simulink model "MS_AEB_201223"  (R2019b)
settings: Solver=ode1  StartTime=0.0  StopTime=inf  FixedStep=0.001  RelTol=1e-3
PreLoadFcn:
  | vehicle = 'Car'; if ~length(which('cmself')), cmenv; end
  | MS_AEB_201223_bus
InitFcn:
  | vehicle = 'Car'; if ~length(which('cmself')), cmenv; end
  | MS_AEB_201223_bus
libraries: CarMaker4SL x4
Description:
  | CarMaker Plug-in Model Target
settings Model: Creator=ambl  LastModifiedBy=ambl
settings RTWCC: Description=CarMaker Plug-in Model Target  SystemTargetFile=CarMaker.tlc  TemplateMakefile=CarMaker_unix-linux64.tmf
settings CodeAppCC: MaxIdLength=127
settings STFCustomTargetCC: TargetLangStandard=C99 (ISO)  CombineOutputUpdateFcns=on  MultiInstanceERTCode=on  CodeInterfacePackaging=Reusable function  GenerateAllocFcn=on  SystemTargetFile=CarMaker.tlc
settings GRTTargetCC: ParMdlRefBuildCompliant=off  CompOptLevelCompliant=off  ConcurrentExecutionCompliant=off  MatFileLogging=off  MultiInstanceERTCode=on  CodeInterfacePackaging=Reusable function  CPPClassGenCompliant=off  GenerateAllocFcn=on  UseToolchainInfoCompliant=off

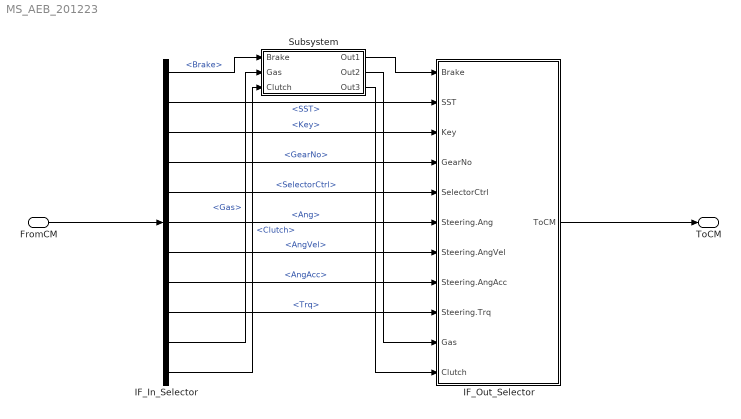
== system MS_AEB_201223 ==
  FromCM : Inport  OutDataTypeStr=Bus: cmVehicleControlIn
  IF_In_Selector : BusSelector  OutputSignals=Brake,SST,Key,GearNo,SelectorCtrl,Steering.Ang,Steering.AngVel,Steering.AngAcc,Steering.Trq,Gas,Clutch
  IF_Out_Selector : Subsystem  mask(Signal Selection){}
      mask help: Signal Selection Block
      settings: OpenFcn=cmSignalSelect('SignalSelection_CB',gcb)
  Subsystem : Subsystem
  ToCM : Outport  OutDataTypeStr=Bus: cmVehicleControlOut
  wires:
  IF_Out_Selector/1(ToCM) -> ToCM/1
  IF_In_Selector/8 -> IF_Out_Selector/8(Steering.AngAcc)  "<AngAcc>"
  FromCM/1 -> IF_In_Selector/1
  IF_In_Selector/10 -> Subsystem/2("Gas ")  "<Gas>"
  Subsystem/2(Out2) -> IF_Out_Selector/10(Gas)
  IF_In_Selector/7 -> IF_Out_Selector/7(Steering.AngVel)  "<AngVel>"
  IF_In_Selector/9 -> IF_Out_Selector/9(Steering.Trq)  "<Trq>"
  IF_In_Selector/4 -> IF_Out_Selector/4(GearNo)  "<GearNo>"
  IF_In_Selector/11 -> Subsystem/3("Clutch ")  "<Clutch>"
  Subsystem/3(Out3) -> IF_Out_Selector/11(Clutch)
  Subsystem/1(Out1) -> IF_Out_Selector/1(Brake)
  IF_In_Selector/5 -> IF_Out_Selector/5(SelectorCtrl)  "<SelectorCtrl>"
  IF_In_Selector/3 -> IF_Out_Selector/3(Key)  "<Key>"
  IF_In_Selector/1 -> Subsystem/1(Brake)  "<Brake>"
  IF_In_Selector/2 -> IF_Out_Selector/2(SST)  "<SST>"
  IF_In_Selector/6 -> IF_Out_Selector/6(Steering.Ang)  "<Ang>"

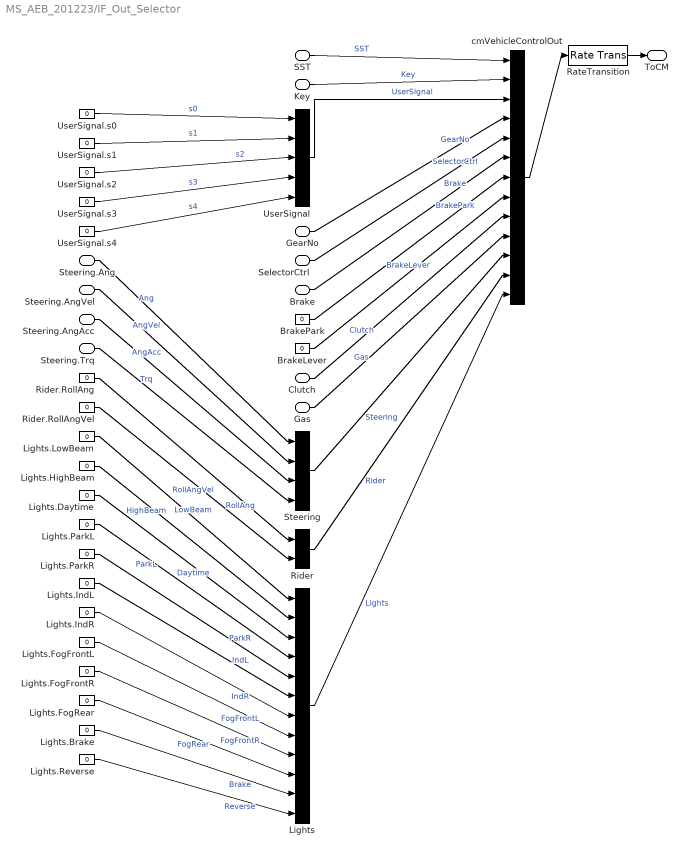
== system MS_AEB_201223/IF_Out_Selector ==
  Brake : Inport
  SST : Inport  Port=2
  Key : Inport  Port=3
  GearNo : Inport  Port=4
  SelectorCtrl : Inport  Port=5
  Steering.Ang : Inport  Port=6
  Steering.AngVel : Inport  Port=7
  Steering.AngAcc : Inport  Port=8
  Steering.Trq : Inport  Port=9
  Gas : Inport  Port=10
  Clutch : Inport  Port=11
  BrakeLever : Constant  Value=0
  BrakePark : Constant  Value=0
  Lights : BusCreator  Inputs=12
  Lights.Brake : Constant  Value=0
  Lights.Daytime : Constant  Value=0
  Lights.FogFrontL : Constant  Value=0
  Lights.FogFrontR : Constant  Value=0
  Lights.FogRear : Constant  Value=0
  Lights.HighBeam : Constant  Value=0
  Lights.IndL : Constant  Value=0
  Lights.IndR : Constant  Value=0
  Lights.LowBeam : Constant  Value=0
  Lights.ParkL : Constant  Value=0
  Lights.ParkR : Constant  Value=0
  Lights.Reverse : Constant  Value=0
  RateTransition : RateTransition  OutPortSampleTime=str2num(get_param(bdroot,'FixedStep'))
  Rider : BusCreator  Inputs=2
  Rider.RollAng : Constant  Value=0
  Rider.RollAngVel : Constant  Value=0
  Steering : BusCreator  Inputs=4
  UserSignal : BusCreator  Inputs=5
  UserSignal.s{0..4} (5 alike) : Constant  Value=0
  cmVehicleControlOut : BusCreator  Inputs=13
  ToCM : Outport
  wires:
  RateTransition/1 -> ToCM/1
  cmVehicleControlOut/1 -> RateTransition/1
  UserSignal/1 -> cmVehicleControlOut/3  "UserSignal"
  UserSignal.s0/1 -> UserSignal/1  "s0"
  UserSignal.s1/1 -> UserSignal/2  "s1"
  UserSignal.s2/1 -> UserSignal/3  "s2"
  UserSignal.s3/1 -> UserSignal/4  "s3"
  UserSignal.s4/1 -> UserSignal/5  "s4"
  BrakePark/1 -> cmVehicleControlOut/7  "BrakePark"
  BrakeLever/1 -> cmVehicleControlOut/8  "BrakeLever"
  Steering/1 -> cmVehicleControlOut/11  "Steering"
  Rider/1 -> cmVehicleControlOut/12  "Rider"
  Rider.RollAng/1 -> Rider/1  "RollAng"
  Rider.RollAngVel/1 -> Rider/2  "RollAngVel"
  Lights/1 -> cmVehicleControlOut/13  "Lights"
  Lights.LowBeam/1 -> Lights/1  "LowBeam"
  Lights.HighBeam/1 -> Lights/2  "HighBeam"
  Lights.Daytime/1 -> Lights/3  "Daytime"
  Lights.ParkL/1 -> Lights/4  "ParkL"
  Lights.ParkR/1 -> Lights/5  "ParkR"
  Lights.IndL/1 -> Lights/6  "IndL"
  Lights.IndR/1 -> Lights/7  "IndR"
  Lights.FogFrontL/1 -> Lights/8  "FogFrontL"
  Lights.FogFrontR/1 -> Lights/9  "FogFrontR"
  Lights.FogRear/1 -> Lights/10  "FogRear"
  Lights.Brake/1 -> Lights/11  "Brake"
  Lights.Reverse/1 -> Lights/12  "Reverse"
  Brake/1 -> cmVehicleControlOut/6  "Brake"
  SST/1 -> cmVehicleControlOut/1  "SST"
  Key/1 -> cmVehicleControlOut/2  "Key"
  GearNo/1 -> cmVehicleControlOut/4  "GearNo"
  SelectorCtrl/1 -> cmVehicleControlOut/5  "SelectorCtrl"
  Steering.Ang/1 -> Steering/1  "Ang"
  Steering.AngVel/1 -> Steering/2  "AngVel"
  Steering.AngAcc/1 -> Steering/3  "AngAcc"
  Steering.Trq/1 -> Steering/4  "Trq"
  Clutch/1 -> cmVehicleControlOut/9  "Clutch"
  Gas/1 -> cmVehicleControlOut/10  "Gas"

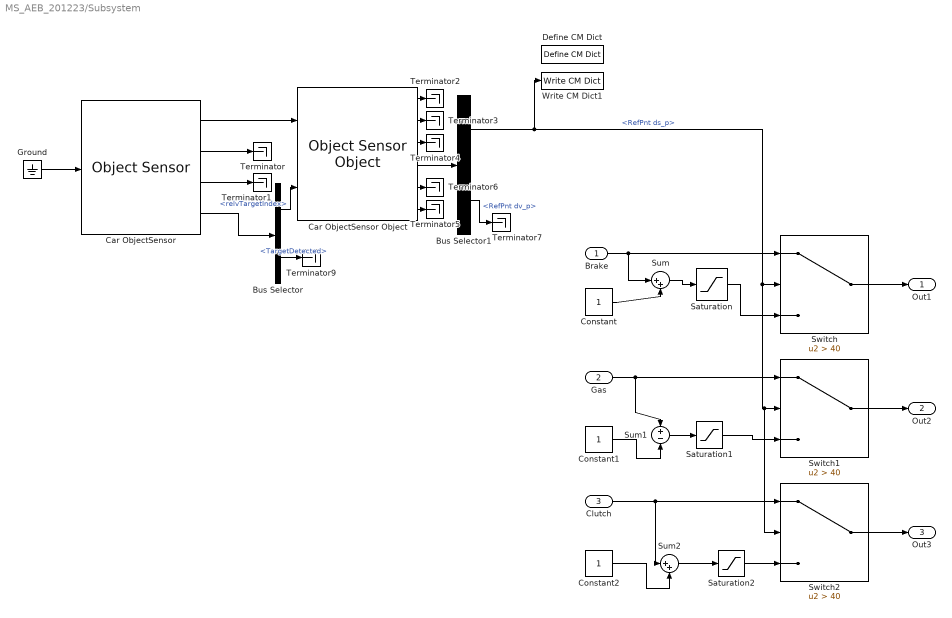
== system MS_AEB_201223/Subsystem ==
  Brake : Inport
  "Gas " : Inport  Port=2
  "Clutch " : Inport  Port=3
  Bus Selector : BusSelector  OutputSignals=relvTargetIndex,TargetDetected
  Bus Selector1 : BusSelector  OutputSignals=RefPnt ds_p,RefPnt dv_p
  Car ObjectSensor : CarMaker4SL/Sensors/Object Sensor  xname=OB00  xstime=Continuous
      settings: SourceProductName=CarMaker4SL
  Car ObjectSensor Object : CarMaker4SL/Sensors/Object Sensor Object  xname=INPORT  ximode=World Objects  xstime=Continuous
      settings: SourceProductName=CarMaker4SL
  Constant : Constant
  Constant1 : Constant
  Constant2 : Constant
  Define CM Dict : CarMaker4SL/Define CM Dict  xname=MS_Quant  xmono=off  xtype=Double4  xdvaplace=None  xnstates=0  xfirststate=0  xinitial=0
  Ground : Ground
  Saturation : Saturate  UpperLimit=1  LowerLimit=0
  Saturation1 : Saturate  UpperLimit=1  LowerLimit=0
  Saturation2 : Saturate  UpperLimit=1  LowerLimit=0
  Sum : Sum  Inputs=|++
  Sum1 : Sum  Inputs=+-
  Sum2 : Sum  Inputs=|++
  Switch : Switch  Criteria=u2 > Threshold  Threshold=40
  Switch1 : Switch  Criteria=u2 > Threshold  Threshold=40
  Switch2 : Switch  Criteria=u2 > Threshold  Threshold=40
  Terminator{,1..7,9} (9 alike) : Terminator
  Write CM Dict1 : CarMaker4SL/Write CM Dict  xname=MS_Quant  xsync=off
  Out1 : Outport
  Out2 : Outport  Port=2
  Out3 : Outport  Port=3
  wires:
  Car ObjectSensor/1 -> Car ObjectSensor Object/1
  Bus Selector1/1 -> Switch2/2, Switch1/2, Switch/2, Write CM Dict1/1  "<RefPnt ds_p>"
  Brake/1 -> Sum/1, Switch/1
  Car ObjectSensor Object/3 -> Terminator4/1
  Car ObjectSensor/3 -> Terminator1/1
  Car ObjectSensor Object/6 -> Terminator5/1
  Car ObjectSensor Object/5 -> Terminator6/1
  Car ObjectSensor Object/1 -> Terminator2/1
  Ground/1 -> Car ObjectSensor/1
  Sum/1 -> Saturation/1
  Bus Selector/1 -> Car ObjectSensor Object/2  "<relvTargetIndex>"
  Car ObjectSensor/2 -> Terminator/1
  Switch/1 -> Out1/1
  Car ObjectSensor Object/4 -> Bus Selector1/1
  Car ObjectSensor/4 -> Bus Selector/1
  Bus Selector1/2 -> Terminator7/1  "<RefPnt dv_p>"
  Car ObjectSensor Object/2 -> Terminator3/1
  Bus Selector/2 -> Terminator9/1  "<TargetDetected>"
  Constant/1 -> Sum/2
  Switch1/1 -> Out2/1
  "Gas "/1 -> Sum1/1, Switch1/1
  Sum1/1 -> Saturation1/1
  Constant1/1 -> Sum1/2
  Switch2/1 -> Out3/1
  Constant2/1 -> Sum2/2
  Sum2/1 -> Saturation2/1
  "Clutch "/1 -> Sum2/1, Switch2/1
  Saturation/1 -> Switch/3
  Saturation1/1 -> Switch1/3
  Saturation2/1 -> Switch2/3
